simulink model "lab1_pre_simulink_"  (R2025a)
settings: Solver=ode1  StartTime=0.0  StopTime=4  FixedStep=0.002  RelTol=1e-3
values from neighbouring files (symbols this model uses):
  fc = 45    [prelab1_new.m]
  WindowSize = 5    [prelab1_new.m]
  zeta = 0.707    [prelab1_new.m]
settings Model: Creator=alexj  LastModifiedBy=alexj

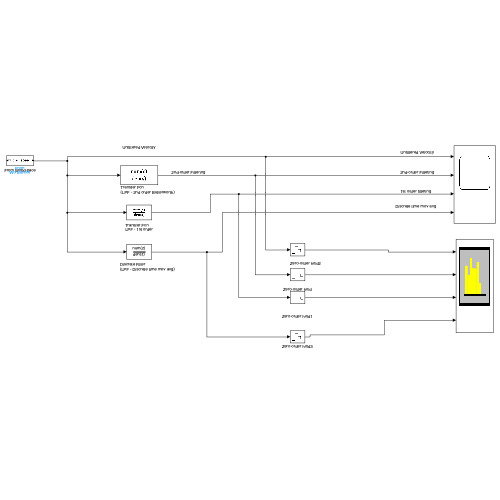
[thumbnail: Simulink's stored preview of the top-level diagram]
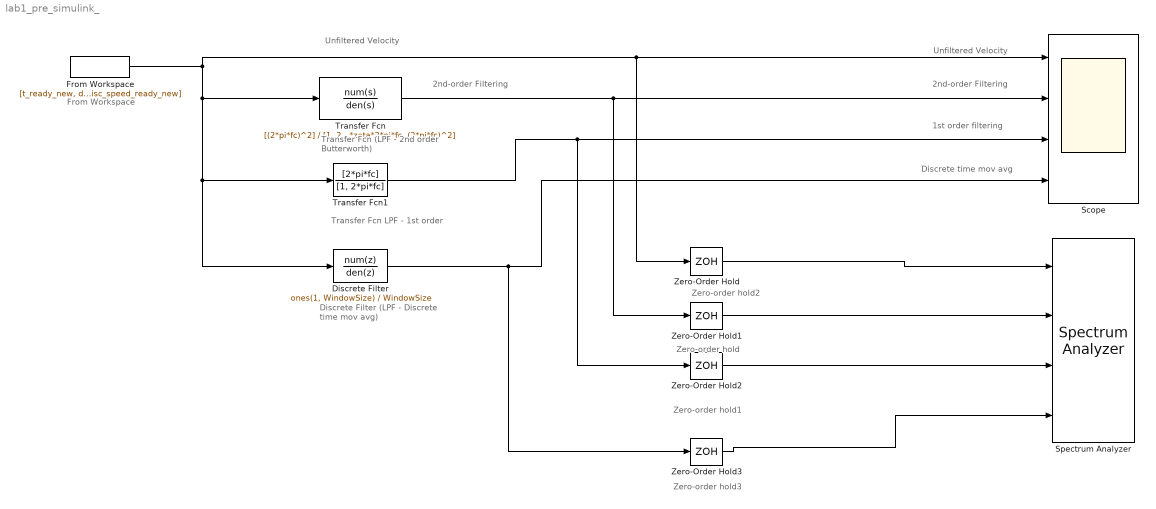
== system lab1_pre_simulink_ ==
  note: Discrete Filter
      | (LPF - Discrete time mov avg)
  note: Transfer Fcn
      | LPF - 1st order
  note: Transfer Fcn
      | (LPF - 2nd order Butterworth)
  note: 2nd-order Filtering
  note: Unfiltered Velocity
  note: From Workspace
  note: Zero-order hold2
  note: Zero-order hold
  note: Zero-order hold1
  note: Zero-order hold3
  note: Unfiltered Velocity
  note: 2nd-order Filtering
  note: 1st order filtering
  note: Discrete time mov avg
  Discrete Filter : DiscreteFilter  Numerator=ones(1, WindowSize)  Denominator=WindowSize
  From Workspace : FromWorkspace  VariableName=[t_ready_new, disc_speed_ready_new]
  Scope : Scope  NumInputPorts=4
      settings: ActiveDisplayYMinimum=-222.27093209154054  ActiveDisplayYMaximum=206.96923115382941
  Spectrum Analyzer : SpectrumAnalyzer  NumInputPorts=4  WindowPosition=[639.000000,178.000000,800.000000,500.000000,]  ScopeFrameLocation=window  WindowInvariantSamplesPerUpdate=on  YLimits=[-37.8164 71.0539]
  Transfer Fcn : TransferFcn  Numerator=[(2*pi*fc)^2]  Denominator=[1, 2*zeta*2*pi*fc, (2*pi*fc)^2]
  Transfer Fcn1 : TransferFcn  Numerator=[2*pi*fc]  Denominator=[1, 2*pi*fc]
  Zero-Order Hold{,1..3} (4 alike) : ZeroOrderHold  SampleTime=-1
  wires:
  From Workspace/1 -> Discrete Filter/1, Transfer Fcn1/1, Transfer Fcn/1, Zero-Order Hold/1, Scope/1
  Transfer Fcn/1 -> Zero-Order Hold1/1, Scope/2
  Zero-Order Hold/1 -> Spectrum Analyzer/1
  Zero-Order Hold1/1 -> Spectrum Analyzer/2
  Transfer Fcn1/1 -> Zero-Order Hold2/1, Scope/3
  Discrete Filter/1 -> Zero-Order Hold3/1, Scope/4
  Zero-Order Hold2/1 -> Spectrum Analyzer/3
  Zero-Order Hold3/1 -> Spectrum Analyzer/4
